simulink model "stanleySimple"  (R2020b)
settings: Solver=VariableStepAuto  StartTime=0.0  StopTime=inf  FixedStep=0.001  RelTol=1e-3
PreLoadFcn:
  | setUpModel
  | close
model workspace (MAT data in the model file):
  firstWarning = 0
  originalScenarioChecksum = 'F73A6DA3C723D3CA73A6F931B7A52A9C'
undefined symbols (not defined in the file or in its folder): curvature, direction, gradbp, psi_o, thetaRefs, velt_res, X_o, xRef2s, Y_o, yRef2s
libraries: vehdynlibviscommon x1, simulink_extras x1, drivingvehiclecontroller x1, autolibshared x1
settings Model: PacingRate=0.700000  Creator=valakshe  LastModifiedBy=valakshe

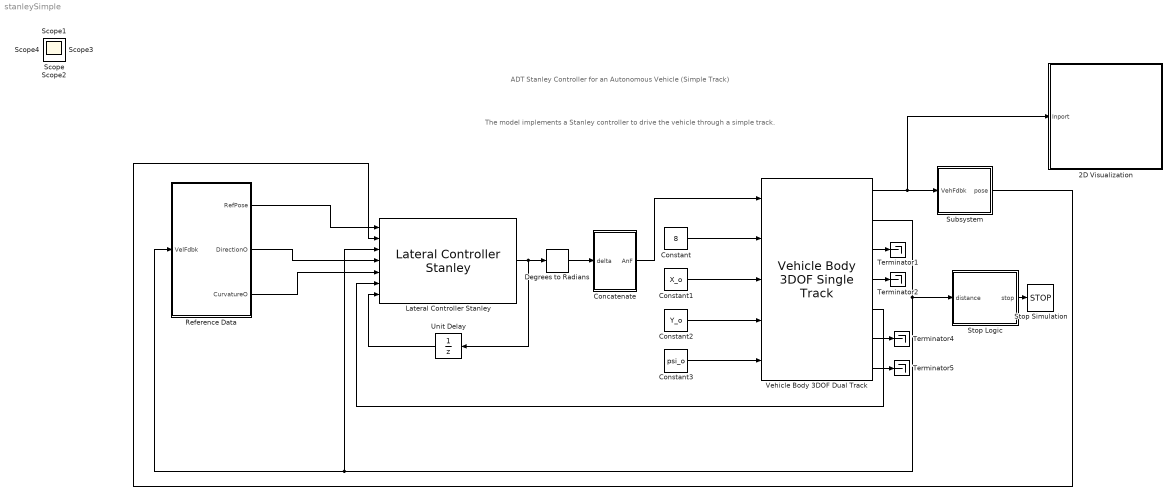
== system stanleySimple ==
  note: ADT Stanley Controller for an Autonomous Vehicle
      | (Simple Track)
  note: The model implements a Stanley controller to drive the vehicle through a simple track.
  2D Visualization : Subsystem
      mask Display: image("visualization.JPG");
  Concatenate : Subsystem
  Constant : Constant  Value=8
  Constant1 : Constant  Value=X_o
  Constant2 : Constant  Value=Y_o
  Constant3 : Constant  Value=psi_o
  Degrees to Radians : simulink_extras/Transformations/Degrees to Radians
  Lateral Controller Stanley : drivingvehiclecontroller/Lateral Controller Stanley  ModelType=Dynamic bicycle model  PositionGainF=2.5  PositionGainR=2.5  YawRateGain=0.2  DelayGain=0.2  VehicleMass=2000  Lf=1.4  Lr=1.6  TireStiffness=12e3  Wheelbase=3  MaxSteeringAngle=35
      settings: SourceProductBaseCode=DR
  Reference Data : Subsystem  VariantControl=Stanley
  Stop Logic : Subsystem
  Stop Simulation : Stop
  Subsystem : Subsystem
  Terminator{1..2,4..5} (4 alike) : Terminator
  Unit Delay : UnitDelay  SampleTime=-1  HasFrameUpgradeWarning=on
  Vehicle Body 3DOF Dual Track : autolibshared/Vehicle Body 3DOF Single Track  trackMode=Dual  inputMode=External longitudinal velocity  frontSteerMode=on  rearSteerMode=off  windMode=off  muMode=off  extFMode=off  extMMode=off  htchFMode=off  htchMMode=off  extXo=on  extpsio=on  extxdoto=off  extro=off  extYo=on  extTamb=off  extydoto=off  aMode=2  NF=2  NR=2  m=2000  a=1.4  b=1.6  h=0.35  dh=1  hh=0.2  X_o=0  xdot_o=velt_res(1)  CalphaMode=off  sigmaMode=on  d=0  hl=0  w=[1.4,1.4]  Cy_f=12e3  Cy_r=11e3  sigma_f=.1  sigma_r=.1  alpha_f_brk=[-.1 .1]  Cy_f_data=[-9e3 9e3]  alpha_r_brk=[-.1 .1]  Cy_r_data=[-9e3 9e3]  Y_o=0  ydot_o=0  Izz=4000  psi_o=0  r_o=0  Af=2  Cd=.3  Cl=.1  Cpm=.1  beta_w=[0:0.01:0.3]  Cs=[0:0.03:0.9]  Cym=[0:0.01:0.3]  Pabs=101325  Tair=273  g=9.81  mu=1  xdot_tol=.01  Fznom=5000  Fxtire_sat=7e4  Fytire_sat=7e4  longOff=0  latOff=0  vertOff=0  wrapAng=off
      settings: SourceProductBaseCode=PW,DR,MT,UV,VE
  Scope{,1..4} (5 alike) : Scope
  wires:
  Constant3/1 -> Vehicle Body 3DOF Dual Track/5
  Constant2/1 -> Vehicle Body 3DOF Dual Track/4
  Constant1/1 -> Vehicle Body 3DOF Dual Track/3
  Constant/1 -> Vehicle Body 3DOF Dual Track/2
  Vehicle Body 3DOF Dual Track/1 -> Subsystem/1(VehFdbk), 2D Visualization/1(Inport)
  Reference Data/2(DirectionO) -> Lateral Controller Stanley/4
  Lateral Controller Stanley/1 -> Unit Delay/1, Degrees to Radians/1
  Concatenate/1(AnF) -> Vehicle Body 3DOF Dual Track/1
  Degrees to Radians/1 -> Concatenate/1(delta)
  Vehicle Body 3DOF Dual Track/3 -> Terminator1/1
  Vehicle Body 3DOF Dual Track/4 -> Terminator2/1
  Vehicle Body 3DOF Dual Track/5 -> Lateral Controller Stanley/6
  Vehicle Body 3DOF Dual Track/6 -> Terminator4/1
  Vehicle Body 3DOF Dual Track/7 -> Terminator5/1
  Subsystem/1(pose) -> Lateral Controller Stanley/2
  Reference Data/1(RefPose) -> Lateral Controller Stanley/1
  Reference Data/3(CurvatureO) -> Lateral Controller Stanley/5
  Unit Delay/1 -> Lateral Controller Stanley/7
  Stop Logic/1(stop) -> Stop Simulation/1
  Vehicle Body 3DOF Dual Track/2 -> Stop Logic/1(distance), Lateral Controller Stanley/3, Reference Data/1(VelFdbk)

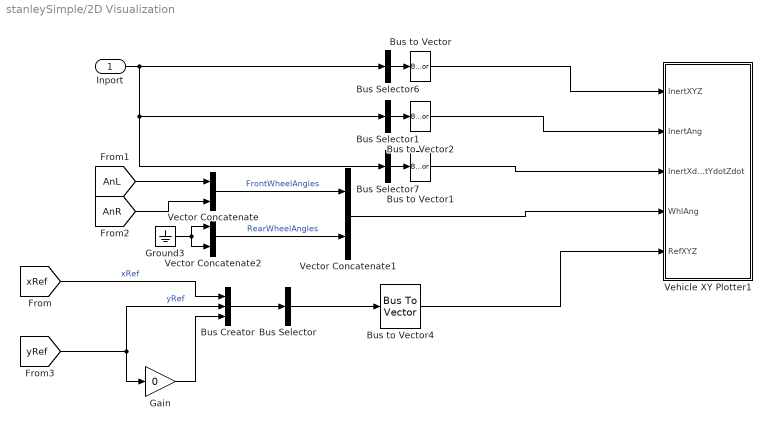
== system stanleySimple/2D Visualization ==
  Inport : Inport
  Bus Creator : BusCreator  Inputs=3
  Bus Selector : BusSelector  OutputSignals=xRef,yRef,signal3  OutputAsBus=on
  Bus Selector1 : BusSelector  OutputSignals=InertFrm.Cg.Ang.phi,InertFrm.Cg.Ang.theta,InertFrm.Cg.Ang.psi  OutputAsBus=on
  Bus Selector6 : BusSelector  OutputSignals=InertFrm.Geom.Disp.X,InertFrm.Geom.Disp.Y,InertFrm.Geom.Disp.Z  OutputAsBus=on
  Bus Selector7 : BusSelector  OutputSignals=InertFrm.Geom.Vel.Xdot,InertFrm.Geom.Vel.Ydot,InertFrm.Geom.Vel.Zdot  OutputAsBus=on
  Bus to Vector{,1..2,4} (4 alike) : BusToVector
  Gain : Gain  Gain=0
  Ground3 : Ground
  Vector Concatenate : Concatenate
  Vector Concatenate1 : Concatenate
  Vector Concatenate2 : Concatenate
  Vehicle XY Plotter1 : Subsystem  mask(Vehicle XY Plotter){extRef=on, extStats=off, extTireF=off, a=2, b=2, w=2, figBorder=10, bufferSize=1024, velNorm=5, tireFNorm=1000, pltDT=0.2}
      mask prompts: extRef "Plot path reference, extRef"; extStats "Display speed, RPM and Gear"; extTireF "Display tire forces"; a "Distance to front axle from CG, a [m]:"; b "Distance to rear axle from CG, b [m]:"; w "Track width, w [m]:"; figBorder "Distance to figure borders, figBorder [m]:"; bufferSize "Path buffer sampe size, bufferSize []:"; velNorm "Velocity vector scaling, velNorm [m*s/m]:"; tireFNorm "Tire force vector scaling, tireFNorm [m/N]:"; pltDT "Plot update rate, pltDT [s]:"
      mask help:
      | This block will display a MATLAB figure which indicates the vehicle path, current position and heading velocity.
      | An optional path reference is also provided.
      mask init:
      | block = gcb;
      | if autoblkschecksimstopped(block)
      |     ParamNames = {'extRef';'extStats';'extTireF';'extTireF'};
      |     PortNames = {'RefXYZ';'Stats';'TireFx';'TireFy'};
      |     for idx=1:length(PortNames)
      |         InportOption  = {'built-in/Ground', [PortNames{idx}, ' Ground'];...
      |             'built-in/Inport',PortNames{idx}};
      |         if ~strcmp(get_param(block,ParamNames{idx}),'on')
      |             NewBlkHdl = autoblksreplaceblock(block, InportOption, 1);
      |             set_param(NewBlkHdl, 'ShowName', 'off');
      |         else
      |             autoblksreplaceblock(block, InportOption, 2);
      |         end
      |     end
      |     InportNames = {'InertXYZ';'InertAng';'InertXdotYdotZdot';'WhlAng';'RefXYZ';'Stats';'TireFx';'TireFy'};
      |     FoundNames = get_param(find_system(block, 'LookUnderMasks', 'all', 'SearchDepth', 1, 'FollowLinks', 'on', 'BlockType', 'Inport'), 'Name');
      |     [~,PortI] = intersect(InportNames, FoundNames);
      |     PortI = sort(PortI);
      |     for idx = 1:length(PortI)
      |         set_param([block, '/', InportNames{PortI(idx)}], 'Port', num2str(idx));
      |     end
      | end
      mask TypeOptions a: Vehicle XY Plotter/a
      mask TypeOptions b: Vehicle XY Plotter/b
      mask TypeOptions w: Vehicle XY Plotter/w
      mask TypeOptions figBorder: Vehicle XY Plotter/figBorder
      mask TypeOptions bufferSize: Vehicle XY Plotter/bufferSize
      mask TypeOptions velNorm: Vehicle XY Plotter/velNorm
      mask TypeOptions tireFNorm: Vehicle XY Plotter/tireFNorm
      mask DialogControl Container3 Prompt: Plot and Display Options
  wires:
  Bus Creator/1 -> Bus Selector/1
  [xRef] -> Bus Creator/1  "xRef"
  Gain/1 -> Bus Creator/3
  [yRef] -> Gain/1, Bus Creator/2  "yRef"
  Bus Selector/1 -> Bus to Vector4/1
  Bus to Vector4/1 -> Vehicle XY Plotter1/5(RefXYZ)
  Inport/1 -> Bus Selector6/1, Bus Selector1/1, Bus Selector7/1
  [AnR] -> Vector Concatenate/2
  Bus Selector1/1 -> Bus to Vector2/1
  Bus to Vector2/1 -> Vehicle XY Plotter1/2(InertAng)
  Bus to Vector/1 -> Vehicle XY Plotter1/1(InertXYZ)
  Bus to Vector1/1 -> Vehicle XY Plotter1/3(InertXdotYdotZdot)
  Bus Selector7/1 -> Bus to Vector1/1
  Vector Concatenate2/1 -> Vector Concatenate1/2  "RearWheelAngles"
  [AnL] -> Vector Concatenate/1
  Vector Concatenate/1 -> Vector Concatenate1/1  "FrontWheelAngles"
  Bus Selector6/1 -> Bus to Vector/1
  Ground3/1 -> Vector Concatenate2/2, Vector Concatenate2/1
  Vector Concatenate1/1 -> Vehicle XY Plotter1/4(WhlAng)

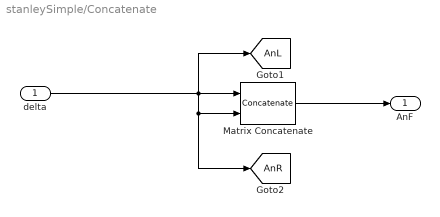
== system stanleySimple/Concatenate ==
  delta : Inport
  Matrix Concatenate : Concatenate
  AnF : Outport  VectorParamsAs1DForOutWhenUnconnected=off
  tag scope: AnL=global, AnR=global
  wires:
  delta/1 -> Matrix Concatenate/1, Matrix Concatenate/2, [AnR], [AnL]
  Matrix Concatenate/1 -> AnF/1

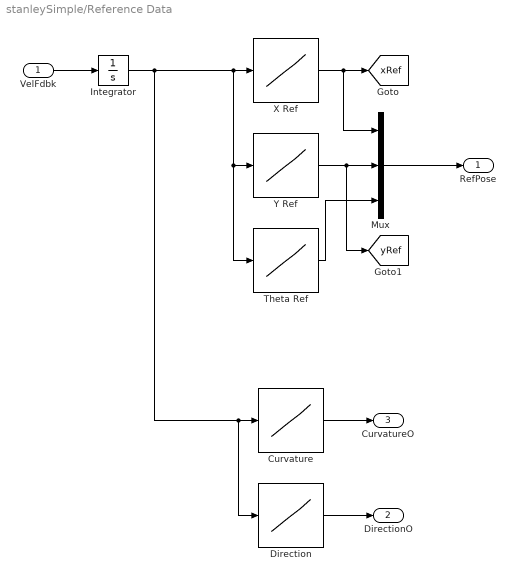
== system stanleySimple/Reference Data ==
  VelFdbk : Inport
  Curvature : Lookup_n-D  NumberOfTableDimensions=1  BreakpointsForDimension1=gradbp  Table=curvature  InternalRulePriority=Speed  RndMeth=Simplest  InputSameDT=on
  Direction : Lookup_n-D  NumberOfTableDimensions=1  BreakpointsForDimension1=gradbp  Table=direction  InternalRulePriority=Speed  RndMeth=Simplest  InputSameDT=on
  Integrator : Integrator
  Mux : Mux  Inputs=3
  Theta Ref : Lookup_n-D  NumberOfTableDimensions=1  BreakpointsForDimension1=gradbp  Table=thetaRefs  InternalRulePriority=Speed  RndMeth=Simplest  InputSameDT=on
  X Ref : Lookup_n-D  NumberOfTableDimensions=1  BreakpointsForDimension1=gradbp  Table=xRef2s  InternalRulePriority=Speed  RndMeth=Simplest  InputSameDT=on
  Y Ref : Lookup_n-D  NumberOfTableDimensions=1  BreakpointsForDimension1=gradbp  Table=yRef2s  InternalRulePriority=Speed  RndMeth=Simplest  InputSameDT=on
  RefPose : Outport
  DirectionO : Outport  Port=2
  CurvatureO : Outport  Port=3
  tag scope: xRef=global, yRef=global
  wires:
  Direction/1 -> DirectionO/1
  Curvature/1 -> CurvatureO/1
  Y Ref/1 -> Mux/2, [yRef]
  Mux/1 -> RefPose/1
  X Ref/1 -> Mux/1, [xRef]
  Theta Ref/1 -> Mux/3
  Integrator/1 -> Curvature/1, Direction/1, Y Ref/1, Theta Ref/1, X Ref/1
  VelFdbk/1 -> Integrator/1

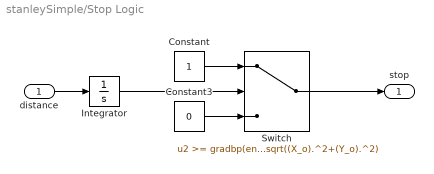
== system stanleySimple/Stop Logic ==
  distance : Inport
  Constant : Constant
  Constant3 : Constant  Value=0
  Integrator : Integrator  InitialCondition=sqrt((X_o).^2+(Y_o).^2)
  Switch : Switch  Threshold=gradbp(end)+sqrt((X_o).^2+(Y_o).^2)
  stop : Outport
  wires:
  Switch/1 -> stop/1
  Constant3/1 -> Switch/3
  distance/1 -> Integrator/1
  Constant/1 -> Switch/1
  Integrator/1 -> Switch/2

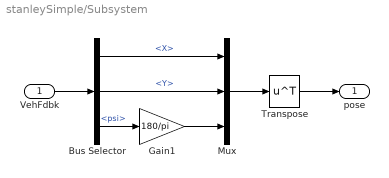
== system stanleySimple/Subsystem ==
  VehFdbk : Inport
  Bus Selector : BusSelector  OutputSignals=InertFrm.Cg.Disp.X,InertFrm.Cg.Disp.Y,InertFrm.Cg.Ang.psi
  Gain1 : Gain  Gain=180/pi
  Mux : Mux  Inputs=3
  Transpose : Math  Operator=transpose  SignedPower=on  SaturateOnIntegerOverflow=on
  pose : Outport
  wires:
  Mux/1 -> Transpose/1
  VehFdbk/1 -> Bus Selector/1
  Bus Selector/1 -> Mux/1  "<X>"
  Gain1/1 -> Mux/3
  Bus Selector/2 -> Mux/2  "<Y>"
  Transpose/1 -> pose/1
  Bus Selector/3 -> Gain1/1  "<psi>"

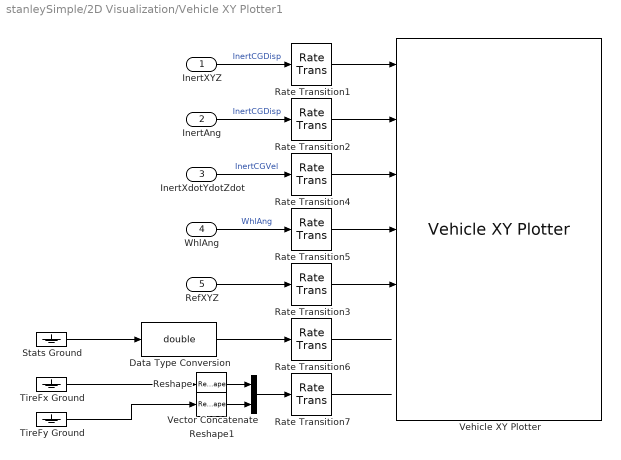
== system stanleySimple/2D Visualization/Vehicle XY Plotter1 ==
  InertXYZ : Inport
  InertAng : Inport  Port=2
  InertXdotYdotZdot : Inport  Port=3
  WhlAng : Inport  Port=4
  RefXYZ : Inport  Port=5
  Data Type Conversion : DataTypeConversion  OutDataTypeStr=double
  Rate Transition{1..7} (7 alike) : RateTransition  Deterministic=off  OutPortSampleTime=pltDT
  Reshape : Reshape  OutputDimensionality=Row vector (2-D)
  Reshape1 : Reshape  OutputDimensionality=Row vector (2-D)
  Stats Ground : Ground
  TireFx Ground : Ground
  TireFy Ground : Ground
  Vector Concatenate : Concatenate  Mode=Multidimensional array
  Vehicle XY Plotter : vehdynlibviscommon/Vehicle XY Plotter  bufferSize=bufferSize  w=w  a=a  b=b  figBorder=figBorder  velNorm=velNorm  tireFNorm=tireFNorm
      settings: SourceProductBaseCode=VE
  wires:
  TireFy Ground/1 -> Reshape1/1
  TireFx Ground/1 -> Reshape/1
  Stats Ground/1 -> Data Type Conversion/1
  InertAng/1 -> Rate Transition2/1  "InertCGDisp"
  InertXdotYdotZdot/1 -> Rate Transition4/1  "InertCGVel"
  InertXYZ/1 -> Rate Transition1/1  "InertCGDisp"
  WhlAng/1 -> Rate Transition5/1  "WhlAng"
  Rate Transition3/1 -> Vehicle XY Plotter/5
  Rate Transition1/1 -> Vehicle XY Plotter/1
  Rate Transition2/1 -> Vehicle XY Plotter/2
  Rate Transition4/1 -> Vehicle XY Plotter/3
  Rate Transition5/1 -> Vehicle XY Plotter/4
  Rate Transition6/1 -> ?
  Data Type Conversion/1 -> Rate Transition6/1
  Rate Transition7/1 -> ?
  RefXYZ/1 -> Rate Transition3/1
  Reshape/1 -> Vector Concatenate/1
  Reshape1/1 -> Vector Concatenate/2
  Vector Concatenate/1 -> Rate Transition7/1
